simulink model "sim_att_dist_obs_tie_2025"  (R2020a)
settings: Solver=ode4  StartTime=0.0  StopTime=30.0  FixedStep=0.01  RelTol=1e-3
values from neighbouring files (symbols this model uses):
  beta_Phi_1 = pp0 * cal_frac_squ( 3, p_p0_plus_1, q_p0_plus_1 )                          * cal_frac_squ( eps_s_bar / pi, p_p0_min_2, q_p0_min_2 )                          / ( 2 * ( 2 * pp0 - 1 ) * tanh( gamma0 * ( eps_s_bar / pi ) / 2 ) )                          - ( cal_frac_squ( 3, p_p0_plus_1, q_p0_plus_1 ) * gamma0 / ( 4 * ( 2 * pp0 -1 ) ) )                          * cal_frac_squ( eps_s_bar / pi, p_p0_min_ ...(+136 chars)    [init_att_dist_obs_tie_2025.m]
  beta_Phi_2 = ( 1 - pp0 ) * cal_frac_squ( 3, p_p0_plus_1, q_p0_plus_1 )                          / ( 2 * ( 1 - 2 * pp0 ) * cal_frac_squ( eps_s_bar / pi, p_p0_0, q_p0_0 ) * tanh( gamma0 * ( eps_s_bar / pi ) / 2 ) )                          - ( cal_frac_squ( 3, p_p0_plus_1, q_p0_plus_1 ) * gamma0 / ( 4 * ( 1 - 2 * pp0 ) ) )                          * cal_frac_squ( eps_s_bar / pi, p_1_min_p0, q_1_min_p0 )          ...(+112 chars)    [init_att_dist_obs_tie_2025.m]
  c1_diff_ui = diag([25; 30; 20])    [init_att_dist_obs_tie_2025.m]
  c2_diff_ui = diag([50; 50; 10])    [init_att_dist_obs_tie_2025.m]
  c3_diff_ui = diag([15; 15; 10])    [init_att_dist_obs_tie_2025.m]
  c_w_1 = diag( [20; 15; 15] )    [init_att_dist_obs_tie_2025.m]
  c_w_2 = diag( [20; 15; 15] )    [init_att_dist_obs_tie_2025.m]
  c_w_3 = diag( [2; 2; 2] )    [init_att_dist_obs_tie_2025.m]
  cS0 = diag( [4.5; 4.5; 4.5] )    [init_att_dist_obs_tie_2025.m]
  dw_aa_t = 0.2 * ones(3, 5) + ( 1.0 - 0.2 ) * rand(3, 5)    [init_att_dist_obs_tie_2025.m]
  dw_ff_t = [ 0.4 * ones(1, 5) + ( 1.0 - 0.4 ) * rand(1, 5);                      0.4 * ones(1, 5) + ( 1.0 - 0.4 ) * rand(1, 5);                      0.2 * ones(1, 5) + ( 0.6 - 0.2 ) * rand(1, 5) ]    [init_att_dist_obs_tie_2025.m]
  dw_phi_t = ( - pi / 2 ) * ones(3, 5) + ( pi / 2 - ( - pi / 2 ) ) * rand(3, 5)    [init_att_dist_obs_tie_2025.m]
  dwci_init = zeros(3,5)    [init_att_dist_obs_tie_2025.m]
  eps_s_bar_div_pi = eps_s_bar / pi    (= 0.03)    [init_att_dist_obs_tie_2025.m]
  gamma0 = 20    [init_att_dist_obs_tie_2025.m]
  Ji = zeros(3,3,NF)    [init_att_dist_obs_tie_2025.m]
  k_J_0 = diag( [1; 1; 1] )    [init_att_dist_obs_tie_2025.m]
  lam1w = [40; 40; 40]    [init_att_dist_obs_tie_2025.m]
  lam2w = [50; 50; 50]    [init_att_dist_obs_tie_2025.m]
  Lamd_diff_ui = 0.8    [init_att_dist_obs_tie_2025.m]
  mu_c_theta = 100    [init_att_dist_obs_tie_2025.m]
  p1w = [1; 1; 1]    [init_att_dist_obs_tie_2025.m]
  pos0 = zeros(3, 1)    [init_att_dist_obs_tie_2025.m]
  pp0 = 8 / 11    (= 0.727272727273)    [init_att_dist_obs_tie_2025.m]
  PZ0 = P0(3)    [init_att_dist_obs_tie_2025.m]
  PZ1 = 10    [init_att_dist_obs_tie_2025.m]
  Qci_init = repmat([1;0;0;0],1,NF)    [init_att_dist_obs_tie_2025.m]
  R0 = 4    [init_att_dist_obs_tie_2025.m]
  R1 = 8    [init_att_dist_obs_tie_2025.m]
  Rci_init = zeros(3,3,NF)    [init_att_dist_obs_tie_2025.m]
  Ri_init = zeros(3,3,NF)    [init_att_dist_obs_tie_2025.m]
  Rx2 = 10    [init_att_dist_obs_tie_2025.m]
  Ry2 = 6    [init_att_dist_obs_tie_2025.m]
  Rz2 = 4    [init_att_dist_obs_tie_2025.m]
  T0 = 0    [init_att_dist_obs_tie_2025.m]
  T1 = tseq1    (= 10)    [init_att_dist_obs_tie_2025.m]
  T2 = tseq1 + tseq12 + tseq2    (= 30)    [init_att_dist_obs_tie_2025.m]
  thr_p_plus_1 = cal_frac_squ( 3, p_p0_plus_1, q_p0_plus_1 )    [init_att_dist_obs_tie_2025.m]
  ui_init = zeros(3,NF)    [init_att_dist_obs_tie_2025.m]
  vel0 = zeros(3, 1)    [init_att_dist_obs_tie_2025.m]
  wci_init = zeros(3,5)    [init_att_dist_obs_tie_2025.m]
  zeta_diff_ui = 0.05    [init_att_dist_obs_tie_2025.m]
undefined symbols (not defined in the file or in its folder): cal_frac_squ, p_2_mu, p_2_p0, p_2mu_1, p_3_2mu, p_beta_w_1, p_beta_w_2, p_mu, p_p0_min_1, p_p0_plus_1, q_2_mu, q_2_p0, q_2mu_1, q_3_2mu, q_beta_w_1, q_beta_w_2, q_mu, q_p0_min_1, q_p0_plus_1, Qei_init, Qi_init, Rei_init, V_Phi_Rei_init, wei_init, wi_init
(part 4 of 4)

== matlab function sim_att_dist_obs_tie_2025/generate angular rate disturbance agent 3 ==
  data: dw_3 output; dw_aa_t input; dw_ff_t input; dw_phi_t input; t input
function dw_3 = fcn(dw_aa_t, dw_ff_t, dw_phi_t, t)
%%%% 姿态动力学方程中的扰动项设置
epsil_t = zeros(3, 1);

for kk = 1:5
    epsil_t = epsil_t + dw_aa_t(:, kk) .* sin( 2 * pi * dw_ff_t(:, kk) * t + dw_phi_t(:, kk) );
end

dw_3 = [ epsil_t(1) + 1.6 * sin( 0.2 * t ) + 2.0 * cos( 0.3 * t ) + 1.4 * sin( 0.5 * t ) ...
                + 4 * exp( -0.1 * t ) * sin( 0.5 * t ) + 3 / ( 1 + exp( -0.2 * ( t - 15 ) ) ); ...
                epsil_t(2) + 1.2 * sin( 0.1 * t ) + 3 * cos( 0.2 * t ) + 0.8 * sin( 0.4 * t ) ...
                + 2 * exp( -0.15 * t ) * cos( 0.6 * t ) + 3 / ( 1 + exp( -0.3 * ( t - 25 ) ) ); ...
                epsil_t(3) + 1.8 * sin( 0.1 * t ) + 1.6 * sin( 0.2 * t ) + 1.6 * cos( 0.3 * t ) ...
                + 4 * exp( -0.05 * t ) * sin( 0.4 * t + pi / 4 ) + 3 / ( 1 + exp( -0.5 * ( t - 20 ) ) ) ];

== matlab function sim_att_dist_obs_tie_2025/generate angular rate disturbance agent 4 ==
  data: dw_4 output; dw_aa_t input; dw_ff_t input; dw_phi_t input; t input
function dw_4 = fcn(dw_aa_t, dw_ff_t, dw_phi_t, t)
%%%% 姿态动力学方程中的扰动项设置
epsil_t = zeros(3, 1);

for kk = 1:5
    epsil_t = epsil_t + dw_aa_t(:, kk) .* sin( 2 * pi * dw_ff_t(:, kk) * t + dw_phi_t(:, kk) );
end

dw_4 = [ epsil_t(1) + 1.6 * sin( 0.2 * t ) + 2.0 * cos( 0.3 * t ) + 1.4 * sin( 0.5 * t ) ...
                + 4 * exp( -0.1 * t ) * sin( 0.5 * t ) + 3 / ( 1 + exp( -0.2 * ( t - 15 ) ) ); ...
                epsil_t(2) + 1.2 * sin( 0.1 * t ) + 3 * cos( 0.2 * t ) + 0.8 * sin( 0.4 * t ) ...
                + 2 * exp( -0.15 * t ) * cos( 0.6 * t ) + 3 / ( 1 + exp( -0.3 * ( t - 25 ) ) ); ...
                epsil_t(3) + 1.8 * sin( 0.1 * t ) + 1.6 * sin( 0.2 * t ) + 1.6 * cos( 0.3 * t ) ...
                + 4 * exp( -0.05 * t ) * sin( 0.4 * t + pi / 4 ) + 3 / ( 1 + exp( -0.5 * ( t - 20 ) ) ) ];

== matlab function sim_att_dist_obs_tie_2025/trans to column56 ==
  data: x input; y output
function y = fcn(x)
y = x(:);

== matlab function sim_att_dist_obs_tie_2025/generate angular rate disturbance agent 5 ==
  data: dw_5 output; dw_aa_t input; dw_ff_t input; dw_phi_t input; t input
function dw_5 = fcn(dw_aa_t, dw_ff_t, dw_phi_t, t)
%%%% 姿态动力学方程中的扰动项设置
epsil_t = zeros(3, 1);

for kk = 1:5
    epsil_t = epsil_t + dw_aa_t(:, kk) .* sin( 2 * pi * dw_ff_t(:, kk) * t + dw_phi_t(:, kk) );
end

dw_5 = [ epsil_t(1) + 1.6 * sin( 0.2 * t ) + 2.0 * cos( 0.3 * t ) + 1.4 * sin( 0.5 * t ) ...
                + 4 * exp( -0.1 * t ) * sin( 0.5 * t ) + 3 / ( 1 + exp( -0.2 * ( t - 15 ) ) ); ...
                epsil_t(2) + 1.2 * sin( 0.1 * t ) + 3 * cos( 0.2 * t ) + 0.8 * sin( 0.4 * t ) ...
                + 2 * exp( -0.15 * t ) * cos( 0.6 * t ) + 3 / ( 1 + exp( -0.3 * ( t - 25 ) ) ); ...
                epsil_t(3) + 1.8 * sin( 0.1 * t ) + 1.6 * sin( 0.2 * t ) + 1.6 * cos( 0.3 * t ) ...
                + 4 * exp( -0.05 * t ) * sin( 0.4 * t + pi / 4 ) + 3 / ( 1 + exp( -0.5 * ( t - 20 ) ) ) ];

== matlab function sim_att_dist_obs_tie_2025/trans to column100 ==
  data: x input; y output
function y = fcn(x)
y = x(:);

== matlab function sim_att_dist_obs_tie_2025/trans to column101 ==
  data: x input; y output
function y = fcn(x)
y = x(:);

== matlab function sim_att_dist_obs_tie_2025/trans to column102 ==
  data: x input; y output
function y = fcn(x)
y = x(:);

== matlab function sim_att_dist_obs_tie_2025/trans to column103 ==
  data: x input; y output
function y = fcn(x)
y = x(:);

== matlab function sim_att_dist_obs_tie_2025/trans to column104 ==
  data: x input; y output
function y = fcn(x)
y = x(:);

== matlab function sim_att_dist_obs_tie_2025/trans to column105 ==
  data: x input; y output
function y = fcn(x)
y = x(:);

== matlab function sim_att_dist_obs_tie_2025/trans to column106 ==
  data: x input; y output
function y = fcn(x)
y = x(:);

== matlab function sim_att_dist_obs_tie_2025/trans to column116 ==
  data: x input; y output
function y = fcn(x)
y = x(:);

== matlab function sim_att_dist_obs_tie_2025/cal abs 17 ==
  data: x input; y output
function y = fcn(x)
y = abs(x(:));

== matlab function sim_att_dist_obs_tie_2025/trans to column118 ==
  data: x input; y output
function y = fcn(x)
y = x(:);

== matlab function sim_att_dist_obs_tie_2025/trans to column119 ==
  data: x input; y output
function y = fcn(x)
y = x(:);

== matlab function sim_att_dist_obs_tie_2025/trans to column120 ==
  data: x input; y output
function y = fcn(x)
y = x(:);

== matlab function sim_att_dist_obs_tie_2025/trans to column121 ==
  data: x input; y output
function y = fcn(x)
y = x(:);

== matlab function sim_att_dist_obs_tie_2025/trans to column122 ==
  data: x input; y output
function y = fcn(x)
y = x(:);

== matlab function sim_att_dist_obs_tie_2025/trans to column123 ==
  data: x input; y output
function y = fcn(x)
y = x(:);

== matlab function sim_att_dist_obs_tie_2025/trans to column124 ==
  data: x input; y output
function y = fcn(x)
y = x(:);

== matlab function sim_att_dist_obs_tie_2025/trans to column125 ==
  data: x input; y output
function y = fcn(x)
y = x(:);

== matlab function sim_att_dist_obs_tie_2025/trans to column61 ==
  data: x input; y output
function y = fcn(x)
y = x(:);

== matlab function sim_att_dist_obs_tie_2025/trans to column62 ==
  data: x input; y output
function y = fcn(x)
y = x(:);

== matlab function sim_att_dist_obs_tie_2025/cal abs 18 ==
  data: x input; y output
function y = fcn(x)
y = abs(x(:));

== matlab function sim_att_dist_obs_tie_2025/trans to column63 ==
  data: x input; y output
function y = fcn(x)
y = x(:);

== matlab function sim_att_dist_obs_tie_2025/trans to column64 ==
  data: x input; y output
function y = fcn(x)
y = x(:);

== matlab function sim_att_dist_obs_tie_2025/trans to column65 ==
  data: x input; y output
function y = fcn(x)
y = x(:);

== matlab function sim_att_dist_obs_tie_2025/trans to column66 ==
  data: x input; y output
function y = fcn(x)
y = x(:);

== matlab function sim_att_dist_obs_tie_2025/trans to column67 ==
  data: x input; y output
function y = fcn(x)
y = x(:);

== matlab function sim_att_dist_obs_tie_2025/trans to column68 ==
  data: x input; y output
function y = fcn(x)
y = x(:);

== matlab function sim_att_dist_obs_tie_2025/trans to column69 ==
  data: x input; y output
function y = fcn(x)
y = x(:);

== matlab function sim_att_dist_obs_tie_2025/trans to column70 ==
  data: x input; y output
function y = fcn(x)
y = x(:);

== matlab function sim_att_dist_obs_tie_2025/trans to column71 ==
  data: x input; y output
function y = fcn(x)
y = x(:);

== matlab function sim_att_dist_obs_tie_2025/trans to column72 ==
  data: x input; y output
function y = fcn(x)
y = x(:);

== matlab function sim_att_dist_obs_tie_2025/cal sig_x1_tilt agent 4 ==
  data: sig_x1_tilt_1_4 output; x1_tilt_vec input; x1_tilt_squ_1_4 input; sig_x1_tilt_2_4 output; x1_tilt_squ_2_4 input; sig_x1_tilt_3_4 output
function [sig_x1_tilt_1_4, sig_x1_tilt_2_4, sig_x1_tilt_3_4] = fcn(x1_tilt_vec, x1_tilt_squ_1_4, x1_tilt_squ_2_4)
%%%% 计算平滑递增函数
iiuav = 4;
sig_x1_tilt_1_4 = x1_tilt_vec(:,iiuav) .* sign(x1_tilt_vec(:,iiuav));
sig_x1_tilt_2_4 = x1_tilt_squ_1_4(:) .* sign(x1_tilt_vec(:,iiuav));
sig_x1_tilt_3_4 = x1_tilt_squ_2_4(:) .* sign(x1_tilt_vec(:,iiuav));

== matlab function sim_att_dist_obs_tie_2025/trans to column73 ==
  data: x input; y output
function y = fcn(x)
y = x(:);

== matlab function sim_att_dist_obs_tie_2025/trans to column74 ==
  data: x input; y output
function y = fcn(x)
y = x(:);

== matlab function sim_att_dist_obs_tie_2025/trans to column75 ==
  data: x input; y output
function y = fcn(x)
y = x(:);

== matlab function sim_att_dist_obs_tie_2025/trans to column76 ==
  data: x input; y output
function y = fcn(x)
y = x(:);

== matlab function sim_att_dist_obs_tie_2025/trans to column77 ==
  data: x input; y output
function y = fcn(x)
y = x(:);

== matlab function sim_att_dist_obs_tie_2025/trans to column78 ==
  data: x input; y output
function y = fcn(x)
y = x(:);

== matlab function sim_att_dist_obs_tie_2025/trans to column79 ==
  data: x input; y output
function y = fcn(x)
y = x(:);

== matlab function sim_att_dist_obs_tie_2025/trans to column80 ==
  data: x input; y output
function y = fcn(x)
y = x(:);

== matlab function sim_att_dist_obs_tie_2025/trans to column81 ==
  data: x input; y output
function y = fcn(x)
y = x(:);

== matlab function sim_att_dist_obs_tie_2025/trans to column82 ==
  data: x input; y output
function y = fcn(x)
y = x(:);

== matlab function sim_att_dist_obs_tie_2025/trans to column83 ==
  data: x input; y output
function y = fcn(x)
y = x(:);

== matlab function sim_att_dist_obs_tie_2025/trans to column84 ==
  data: x input; y output
function y = fcn(x)
y = x(:);

== matlab function sim_att_dist_obs_tie_2025/trans to column85 ==
  data: x input; y output
function y = fcn(x)
y = x(:);

== matlab function sim_att_dist_obs_tie_2025/trans to column86 ==
  data: x input; y output
function y = fcn(x)
y = x(:);

== matlab function sim_att_dist_obs_tie_2025/trans to column87 ==
  data: x input; y output
function y = fcn(x)
y = x(:);

== matlab function sim_att_dist_obs_tie_2025/trans to column88 ==
  data: x input; y output
function y = fcn(x)
y = x(:);

== matlab function sim_att_dist_obs_tie_2025/choose ksi_est_err 17 ==
  data: x input; y output
function y = fcn(x)
iiuav = 4;
y = x(:,iiuav);

== matlab function sim_att_dist_obs_tie_2025/trans to column89 ==
  data: x input; y output
function y = fcn(x)
y = x(:);

== matlab function sim_att_dist_obs_tie_2025/trans to column90 ==
  data: x input; y output
function y = fcn(x)
y = x(:);

== matlab function sim_att_dist_obs_tie_2025/trans to column91 ==
  data: x input; y output
function y = fcn(x)
y = x(:);

== matlab function sim_att_dist_obs_tie_2025/trans to column92 ==
  data: x input; y output
function y = fcn(x)
y = x(:);

== matlab function sim_att_dist_obs_tie_2025/trans to column93 ==
  data: x input; y output
function y = fcn(x)
y = x(:);

== matlab function sim_att_dist_obs_tie_2025/trans to column94 ==
  data: x input; y output
function y = fcn(x)
y = x(:);

== matlab function sim_att_dist_obs_tie_2025/trans to column95 ==
  data: x input; y output
function y = fcn(x)
y = x(:);

== matlab function sim_att_dist_obs_tie_2025/trans to column96 ==
  data: x input; y output
function y = fcn(x)
y = x(:);

== matlab function sim_att_dist_obs_tie_2025/trans to column97 ==
  data: x input; y output
function y = fcn(x)
y = x(:);

== matlab function sim_att_dist_obs_tie_2025/trans to column98 ==
  data: x input; y output
function y = fcn(x)
y = x(:);

== matlab function sim_att_dist_obs_tie_2025/choose ksi_est_err 18 ==
  data: x input; y output
function y = fcn(x)
iiuav = 4;
y = x(:,iiuav);

== matlab function sim_att_dist_obs_tie_2025/trans to column99 ==
  data: x input; y output
function y = fcn(x)
y = x(:);

== matlab function sim_att_dist_obs_tie_2025/wi dynam agent 1 ==
  data: Ji input; dwi_1 output; wi_vec input; taui_vec input; dw_vec input
function dwi_1 = fcn(Ji, wi_vec, taui_vec, dw_vec)
%%%% 更新姿态角速率微分方程
iiuav = 1;
dwi_1 = inv(Ji(:,:,iiuav)) * ( -cal_askew_mat(wi_vec(:,iiuav)) * Ji(:,:,iiuav) * wi_vec(:,iiuav) ... 
                                                + taui_vec(:,iiuav) + dw_vec(:,iiuav) );

end

== matlab function sim_att_dist_obs_tie_2025/wi dynam agent 2 ==
  data: Ji input; dwi_2 output; wi_vec input; taui_vec input; dw_vec input
function dwi_2 = fcn(Ji, wi_vec, taui_vec, dw_vec)
%%%% 更新姿态角速率微分方程
iiuav = 2;
dwi_2 = inv(Ji(:,:,iiuav)) * ( -cal_askew_mat(wi_vec(:,iiuav)) * Ji(:,:,iiuav) * wi_vec(:,iiuav) ... 
                                                + taui_vec(:,iiuav) + dw_vec(:,iiuav) );

end

== matlab function sim_att_dist_obs_tie_2025/wi dynam agent 3 ==
  data: Ji input; dwi_3 output; wi_vec input; taui_vec input; dw_vec input
function dwi_3 = fcn(Ji, wi_vec, taui_vec, dw_vec)
%%%% 更新姿态角速率微分方程
iiuav = 3;
dwi_3 = inv(Ji(:,:,iiuav)) * ( -cal_askew_mat(wi_vec(:,iiuav)) * Ji(:,:,iiuav) * wi_vec(:,iiuav) ...
                                                + taui_vec(:,iiuav) + dw_vec(:,iiuav) );

end

== matlab function sim_att_dist_obs_tie_2025/wi dynam agent 4 ==
  data: Ji input; dwi_4 output; wi_vec input; taui_vec input; dw_vec input
function dwi_4 = fcn(Ji, wi_vec, taui_vec, dw_vec)
%%%% 更新姿态角速率微分方程
iiuav = 4;
dwi_4 = inv(Ji(:,:,iiuav)) * ( -cal_askew_mat(wi_vec(:,iiuav)) * Ji(:,:,iiuav) * wi_vec(:,iiuav) ...
                                                + taui_vec(:,iiuav) + dw_vec(:,iiuav) );

end

== matlab function sim_att_dist_obs_tie_2025/wi dynam agent 5 ==
  data: Ji input; dwi_5 output; wi_vec input; taui_vec input; dw_vec input
function dwi_5 = fcn(Ji, wi_vec, taui_vec, dw_vec)
%%%% 更新姿态角速率微分方程
iiuav = 5;
dwi_5 = inv(Ji(:,:,iiuav)) * ( -cal_askew_mat(wi_vec(:,iiuav)) * Ji(:,:,iiuav) * wi_vec(:,iiuav) ...
                                                + taui_vec(:,iiuav) + dw_vec(:,iiuav) );

end

== matlab function sim_att_dist_obs_tie_2025/combine norminal formation control input ==
  data: ui_1 input; ui_vec output; ui_2 input; ui_3 input; ui_4 input; ui_5 input
function ui_vec = fcn(ui_1, ui_2, ui_3, ui_4, ui_5)
%%%% 合并领导者编队跟踪误差结果
ui_vec = [ui_1(:), ui_2(:), ui_3(:), ui_4(:), ui_5(:)];

== matlab function sim_att_dist_obs_tie_2025/trans to column57 ==
  data: x input; y output
function y = fcn(x)
y = x(:);

== matlab function sim_att_dist_obs_tie_2025/control input generator agent 1 ==
  data: u0 input; ui output
function ui  = fcn(u0)
%%%% 给出领导者参考加速度控制输入
g0 = 9.80663;
e3 = [0;0;1];

ui = g0 * e3 + u0(:);

== matlab function sim_att_dist_obs_tie_2025/control input generator agent 2 ==
  data: u0 input; ui output
function ui  = fcn(u0)
%%%% 给出领导者参考加速度控制输入
g0 = 9.80663;
e3 = [0;0;1];

ui = g0 * e3 + u0(:);

== matlab function sim_att_dist_obs_tie_2025/control input generator agent 3 ==
  data: u0 input; ui output
function ui  = fcn(u0)
%%%% 给出领导者参考加速度控制输入
g0 = 9.80663;
e3 = [0;0;1];

ui = g0 * e3 + u0(:);

== matlab function sim_att_dist_obs_tie_2025/control input generator agent 4 ==
  data: u0 input; ui output
function ui  = fcn(u0)
%%%% 给出领导者参考加速度控制输入
g0 = 9.80663;
e3 = [0;0;1];

ui = g0 * e3 + u0(:);

== matlab function sim_att_dist_obs_tie_2025/control input generator agent 5 ==
  data: u0 input; ui output
function ui  = fcn(u0)
%%%% 给出领导者参考加速度控制输入
g0 = 9.80663;
e3 = [0;0;1];

ui = g0 * e3 + u0(:);

== matlab function sim_att_dist_obs_tie_2025/trans to column58 ==
  data: x input; y output
function y = fcn(x)
y = x(:);

== matlab function sim_att_dist_obs_tie_2025/cal abs 19 ==
  data: x input; y output
function y = fcn(x)
y = abs(x(:));

== matlab function sim_att_dist_obs_tie_2025/cal abs 20 ==
  data: x input; y output
function y = fcn(x)
y = abs(x(:));

== matlab function sim_att_dist_obs_tie_2025/cal sig_x1_tilt agent 5 ==
  data: sig_x1_tilt_1_5 output; x1_tilt_vec input; x1_tilt_squ_1_5 input; sig_x1_tilt_2_5 output; x1_tilt_squ_2_5 input; sig_x1_tilt_3_5 output
function [sig_x1_tilt_1_5, sig_x1_tilt_2_5, sig_x1_tilt_3_5] = fcn(x1_tilt_vec, x1_tilt_squ_1_5, x1_tilt_squ_2_5)
%%%% 计算平滑递增函数
iiuav = 5;
sig_x1_tilt_1_5 = x1_tilt_vec(:,iiuav) .* sign(x1_tilt_vec(:,iiuav));
sig_x1_tilt_2_5 = x1_tilt_squ_1_5(:) .* sign(x1_tilt_vec(:,iiuav));
sig_x1_tilt_3_5 = x1_tilt_squ_2_5(:) .* sign(x1_tilt_vec(:,iiuav));

== matlab function sim_att_dist_obs_tie_2025/choose ksi_est_err 19 ==
  data: x input; y output
function y = fcn(x)
iiuav = 5;
y = x(:,iiuav);

== matlab function sim_att_dist_obs_tie_2025/choose ksi_est_err 20 ==
  data: x input; y output
function y = fcn(x)
iiuav = 5;
y = x(:,iiuav);

== matlab function sim_att_dist_obs_tie_2025/trans to column59 ==
  data: x input; y output
function y = fcn(x)
y = x(:);

== matlab function sim_att_dist_obs_tie_2025/trans to column60 ==
  data: x input; y output
function y = fcn(x)
y = x(:);

== matlab function sim_att_dist_obs_tie_2025/cal x1_hat agent 1 ==
  data: d_x1_hat_1 output; Ji input; lam1w input; wi_vec input; taui_vec input; dw_hat_vec input; sig_x1_tilt_1_vec input; sig_x1_tilt_2_vec input; sig_x1_tilt_3_vec input
function d_x1_hat_1 = fcn(Ji, lam1w, wi_vec, taui_vec, dw_hat_vec, sig_x1_tilt_1_vec, sig_x1_tilt_2_vec, sig_x1_tilt_3_vec)
%%%% 计算平滑递增函数
iiuav = 1;
d_x1_hat_1 = -cal_askew_mat(wi_vec(:,iiuav)) * Ji(:,:,iiuav) * wi_vec(:,iiuav) + taui_vec(:,iiuav) ...
                            + dw_hat_vec(:,iiuav) + lam1w(:) .* (sig_x1_tilt_1_vec(:,iiuav) + sig_x1_tilt_2_vec(:,iiuav) + sig_x1_tilt_3_vec(:,iiuav));

== matlab function sim_att_dist_obs_tie_2025/cal x1_hat agent 2 ==
  data: d_x1_hat_2 output; Ji input; lam1w input; wi_vec input; taui_vec input; dw_hat_vec input; sig_x1_tilt_1_vec input; sig_x1_tilt_2_vec input; sig_x1_tilt_3_vec input
function d_x1_hat_2 = fcn(Ji, lam1w, wi_vec, taui_vec, dw_hat_vec, sig_x1_tilt_1_vec, sig_x1_tilt_2_vec, sig_x1_tilt_3_vec)
%%%% 计算平滑递增函数
iiuav = 2;
d_x1_hat_2 = -cal_askew_mat(wi_vec(:,iiuav)) * Ji(:,:,iiuav) * wi_vec(:,iiuav) + taui_vec(:,iiuav) ...
                            + dw_hat_vec(:,iiuav) + lam1w(:) .* (sig_x1_tilt_1_vec(:,iiuav) + sig_x1_tilt_2_vec(:,iiuav) + sig_x1_tilt_3_vec(:,iiuav));

== matlab function sim_att_dist_obs_tie_2025/cal x1_hat agent 3 ==
  data: d_x1_hat_3 output; Ji input; lam1w input; wi_vec input; taui_vec input; dw_hat_vec input; sig_x1_tilt_1_vec input; sig_x1_tilt_2_vec input; sig_x1_tilt_3_vec input
function d_x1_hat_3 = fcn(Ji, lam1w, wi_vec, taui_vec, dw_hat_vec, sig_x1_tilt_1_vec, sig_x1_tilt_2_vec, sig_x1_tilt_3_vec)
%%%% 计算平滑递增函数
iiuav = 3;
d_x1_hat_3 = -cal_askew_mat(wi_vec(:,iiuav)) * Ji(:,:,iiuav) * wi_vec(:,iiuav) + taui_vec(:,iiuav) ...
                            + dw_hat_vec(:,iiuav) + lam1w(:) .* (sig_x1_tilt_1_vec(:,iiuav) + sig_x1_tilt_2_vec(:,iiuav) + sig_x1_tilt_3_vec(:,iiuav));

== matlab function sim_att_dist_obs_tie_2025/cal x1_hat agent 4 ==
  data: d_x1_hat_4 output; Ji input; lam1w input; wi_vec input; taui_vec input; dw_hat_vec input; sig_x1_tilt_1_vec input; sig_x1_tilt_2_vec input; sig_x1_tilt_3_vec input
function d_x1_hat_4 = fcn(Ji, lam1w, wi_vec, taui_vec, dw_hat_vec, sig_x1_tilt_1_vec, sig_x1_tilt_2_vec, sig_x1_tilt_3_vec)
%%%% 计算平滑递增函数
iiuav = 4;
d_x1_hat_4 = -cal_askew_mat(wi_vec(:,iiuav)) * Ji(:,:,iiuav) * wi_vec(:,iiuav) + taui_vec(:,iiuav) ...
                            + dw_hat_vec(:,iiuav) + lam1w(:) .* (sig_x1_tilt_1_vec(:,iiuav) + sig_x1_tilt_2_vec(:,iiuav) + sig_x1_tilt_3_vec(:,iiuav));

== matlab function sim_att_dist_obs_tie_2025/cal x1_hat agent 5 ==
  data: d_x1_hat_5 output; Ji input; lam1w input; wi_vec input; taui_vec input; dw_hat_vec input; sig_x1_tilt_1_vec input; sig_x1_tilt_2_vec input; sig_x1_tilt_3_vec input
function d_x1_hat_5 = fcn(Ji, lam1w, wi_vec, taui_vec, dw_hat_vec, sig_x1_tilt_1_vec, sig_x1_tilt_2_vec, sig_x1_tilt_3_vec)
%%%% 计算平滑递增函数
iiuav = 5;
d_x1_hat_5 = -cal_askew_mat(wi_vec(:,iiuav)) * Ji(:,:,iiuav) * wi_vec(:,iiuav) + taui_vec(:,iiuav) ...
                            + dw_hat_vec(:,iiuav) + lam1w(:) .* (sig_x1_tilt_1_vec(:,iiuav) + sig_x1_tilt_2_vec(:,iiuav) + sig_x1_tilt_3_vec(:,iiuav));

== matlab function sim_att_dist_obs_tie_2025/cal abs 31 ==
  data: x input; y output
function y = fcn(x)
y = abs(x(:));

== matlab function sim_att_dist_obs_tie_2025/cal abs 32 ==
  data: x input; y output
function y = fcn(x)
y = abs(x(:));

== matlab function sim_att_dist_obs_tie_2025/cal abs 33 ==
  data: x input; y output
function y = fcn(x)
y = abs(x(:));

== matlab function sim_att_dist_obs_tie_2025/cal abs 34 ==
  data: x input; y output
function y = fcn(x)
y = abs(x(:));

== matlab function sim_att_dist_obs_tie_2025/cal sig_x1_tilt other agent 2 ==
  data: sig_x1_tilt_4_2 output; x1_tilt_vec input; x1_tilt_squ_4_2 input; sig_x1_tilt_5_2 output; x1_tilt_squ_5_2 input
function [sig_x1_tilt_4_2, sig_x1_tilt_5_2] = fcn(x1_tilt_vec, x1_tilt_squ_4_2, x1_tilt_squ_5_2)
%%%% 计算平滑递增函数
iiuav = 2;
sig_x1_tilt_4_2 = x1_tilt_squ_4_2(:) .* sign(x1_tilt_vec(:,iiuav));
sig_x1_tilt_5_2 = x1_tilt_squ_5_2(:) .* sign(x1_tilt_vec(:,iiuav));

== matlab function sim_att_dist_obs_tie_2025/choose ksi_est_err 33 ==
  data: x input; y output
function y = fcn(x)
iiuav = 2;
y = x(:,iiuav);

== matlab function sim_att_dist_obs_tie_2025/choose ksi_est_err 34 ==
  data: x input; y output
function y = fcn(x)
iiuav = 2;
y = x(:,iiuav);

== matlab function sim_att_dist_obs_tie_2025/trans to column3 ==
  data: x input; y output
function y = fcn(x)
y = x(:);

== matlab function sim_att_dist_obs_tie_2025/trans to column4 ==
  data: x input; y output
function y = fcn(x)
y = x(:);

== matlab function sim_att_dist_obs_tie_2025/cal abs 35 ==
  data: x input; y output
function y = fcn(x)
y = abs(x(:));

== matlab function sim_att_dist_obs_tie_2025/cal abs 36 ==
  data: x input; y output
function y = fcn(x)
y = abs(x(:));

== matlab function sim_att_dist_obs_tie_2025/cal x1_tilt ==
  data: Ji input; p1w input; x1_tilt_vec output; wi_vec input; x1_hat_vec input
function x1_tilt_vec = fcn(Ji, p1w, wi_vec, x1_hat_vec)
%%%% 计算姿态角速率观测误差
x1_tilt_vec = zeros(3,5);
for iiuav = 1:5
    x1_tilt_vec(:,iiuav) = (1 ./ p1w) .* ( Ji(:,:,iiuav) * wi_vec(:,iiuav) - x1_hat_vec(:,iiuav) );
end

== matlab function sim_att_dist_obs_tie_2025/cal sig_x1_tilt other agent 1 ==
  data: sig_x1_tilt_4_1 output; x1_tilt_vec input; x1_tilt_squ_4_1 input; sig_x1_tilt_5_1 output; x1_tilt_squ_5_1 input
function [sig_x1_tilt_4_1, sig_x1_tilt_5_1] = fcn(x1_tilt_vec, x1_tilt_squ_4_1, x1_tilt_squ_5_1)
%%%% 计算平滑递增函数
iiuav = 1;
sig_x1_tilt_4_1 = x1_tilt_squ_4_1(:) .* sign(x1_tilt_vec(:,iiuav));
sig_x1_tilt_5_1 = x1_tilt_squ_5_1(:) .* sign(x1_tilt_vec(:,iiuav));

== matlab function sim_att_dist_obs_tie_2025/cal sig_x1_tilt other agent 3 ==
  data: sig_x1_tilt_4_3 output; x1_tilt_vec input; x1_tilt_squ_4_3 input; sig_x1_tilt_5_3 output; x1_tilt_squ_5_3 input
function [sig_x1_tilt_4_3, sig_x1_tilt_5_3] = fcn(x1_tilt_vec, x1_tilt_squ_4_3, x1_tilt_squ_5_3)
%%%% 计算平滑递增函数
iiuav = 3;
sig_x1_tilt_4_3 = x1_tilt_squ_4_3(:) .* sign(x1_tilt_vec(:,iiuav));
sig_x1_tilt_5_3 = x1_tilt_squ_5_3(:) .* sign(x1_tilt_vec(:,iiuav));

== matlab function sim_att_dist_obs_tie_2025/choose ksi_est_err 35 ==
  data: x input; y output
function y = fcn(x)
iiuav = 3;
y = x(:,iiuav);

== matlab function sim_att_dist_obs_tie_2025/choose ksi_est_err 36 ==
  data: x input; y output
function y = fcn(x)
iiuav = 3;
y = x(:,iiuav);

== matlab function sim_att_dist_obs_tie_2025/choose ksi_est_err 31 ==
  data: x input; y output
function y = fcn(x)
iiuav = 1;
y = x(:,iiuav);

== matlab function sim_att_dist_obs_tie_2025/choose ksi_est_err 32 ==
  data: x input; y output
function y = fcn(x)
iiuav = 1;
y = x(:,iiuav);

== matlab function sim_att_dist_obs_tie_2025/trans to column5 ==
  data: x input; y output
function y = fcn(x)
y = x(:);

== matlab function sim_att_dist_obs_tie_2025/trans to column6 ==
  data: x input; y output
function y = fcn(x)
y = x(:);

== matlab function sim_att_dist_obs_tie_2025/cal abs 37 ==
  data: x input; y output
function y = fcn(x)
y = abs(x(:));

== matlab function sim_att_dist_obs_tie_2025/cal abs 38 ==
  data: x input; y output
function y = fcn(x)
y = abs(x(:));

== matlab function sim_att_dist_obs_tie_2025/cal sig_x1_tilt other agent 4 ==
  data: sig_x1_tilt_4_4 output; x1_tilt_vec input; x1_tilt_squ_4_4 input; sig_x1_tilt_5_4 output; x1_tilt_squ_5_4 input
function [sig_x1_tilt_4_4, sig_x1_tilt_5_4] = fcn(x1_tilt_vec, x1_tilt_squ_4_4, x1_tilt_squ_5_4)
%%%% 计算平滑递增函数
iiuav = 4;
sig_x1_tilt_4_4 = x1_tilt_squ_4_4(:) .* sign(x1_tilt_vec(:,iiuav));
sig_x1_tilt_5_4 = x1_tilt_squ_5_4(:) .* sign(x1_tilt_vec(:,iiuav));

== matlab function sim_att_dist_obs_tie_2025/choose ksi_est_err 37 ==
  data: x input; y output
function y = fcn(x)
iiuav = 4;
y = x(:,iiuav);

== matlab function sim_att_dist_obs_tie_2025/choose ksi_est_err 38 ==
  data: x input; y output
function y = fcn(x)
iiuav = 4;
y = x(:,iiuav);

== matlab function sim_att_dist_obs_tie_2025/trans to column7 ==
  data: x input; y output
function y = fcn(x)
y = x(:);

== matlab function sim_att_dist_obs_tie_2025/combine sig_x1_tilt other ==
  data: sig_x1_tilt_4_1 input; sig_x1_tilt_4_2 input; sig_x1_tilt_4_3 input; sig_x1_tilt_4_4 input; sig_x1_tilt_4_5 input; sig_x1_tilt_4_vec output; sig_x1_tilt_5_1 input; sig_x1_tilt_5_vec output; sig_x1_tilt_5_2 input; sig_x1_tilt_5_3 input; sig_x1_tilt_5_4 input; sig_x1_tilt_5_5 input
function [sig_x1_tilt_4_vec, sig_x1_tilt_5_vec]  = fcn(sig_x1_tilt_4_1, sig_x1_tilt_4_2, sig_x1_tilt_4_3, sig_x1_tilt_4_4, sig_x1_tilt_4_5, ...
                                                                                                                                sig_x1_tilt_5_1, sig_x1_tilt_5_2, sig_x1_tilt_5_3, sig_x1_tilt_5_4, sig_x1_tilt_5_5)
%%%% 合并领导者位置观测器输出结果
sig_x1_tilt_4_vec = [sig_x1_tilt_4_1(:), sig_x1_tilt_4_2(:), sig_x1_tilt_4_3(:), sig_x1_tilt_4_4(:), sig_x1_tilt_4_5(:)];
sig_x1_tilt_5_vec = [sig_x1_tilt_5_1(:), sig_x1_tilt_5_2(:), sig_x1_tilt_5_3(:), sig_x1_tilt_5_4(:), sig_x1_tilt_5_5(:)];

== matlab function sim_att_dist_obs_tie_2025/trans to column1 ==
  data: x input; y output
function y = fcn(x)
y = x(:);

== matlab function sim_att_dist_obs_tie_2025/trans to column2 ==
  data: x input; y output
function y = fcn(x)
y = x(:);

== matlab function sim_att_dist_obs_tie_2025/trans to column8 ==
  data: x input; y output
function y = fcn(x)
y = x(:);

== matlab function sim_att_dist_obs_tie_2025/cal abs 39 ==
  data: x input; y output
function y = fcn(x)
y = abs(x(:));

== matlab function sim_att_dist_obs_tie_2025/cal abs 40 ==
  data: x input; y output
function y = fcn(x)
y = abs(x(:));

== matlab function sim_att_dist_obs_tie_2025/cal sig_x1_tilt other agent 5 ==
  data: sig_x1_tilt_4_5 output; x1_tilt_vec input; x1_tilt_squ_4_5 input; sig_x1_tilt_5_5 output; x1_tilt_squ_5_5 input
function [sig_x1_tilt_4_5, sig_x1_tilt_5_5] = fcn(x1_tilt_vec, x1_tilt_squ_4_5, x1_tilt_squ_5_5)
%%%% 计算平滑递增函数
iiuav = 5;
sig_x1_tilt_4_5 = x1_tilt_squ_4_5(:) .* sign(x1_tilt_vec(:,iiuav));
sig_x1_tilt_5_5 = x1_tilt_squ_5_5(:) .* sign(x1_tilt_vec(:,iiuav));

== matlab function sim_att_dist_obs_tie_2025/choose ksi_est_err 39 ==
  data: x input; y output
function y = fcn(x)
iiuav = 5;
y = x(:,iiuav);

== matlab function sim_att_dist_obs_tie_2025/choose ksi_est_err 40 ==
  data: x input; y output
function y = fcn(x)
iiuav = 5;
y = x(:,iiuav);

== matlab function sim_att_dist_obs_tie_2025/trans to column9 ==
  data: x input; y output
function y = fcn(x)
y = x(:);

== matlab function sim_att_dist_obs_tie_2025/trans to column10 ==
  data: x input; y output
function y = fcn(x)
y = x(:);

== matlab function sim_att_dist_obs_tie_2025/cal neso dw_hat agent 2 ==
  data: lam2w input; p1w input; sig_x1_tilt_1_vec input; sig_x1_tilt_4_vec input; sig_x1_tilt_5_vec input; d_dw_hat_2 output
function d_dw_hat_2 = fcn(lam2w, p1w, sig_x1_tilt_1_vec, sig_x1_tilt_4_vec, sig_x1_tilt_5_vec)
%%%% 计算扰动观测值
iiuav = 2;
d_dw_hat_2 = (lam2w(:) ./ p1w(:)) .* (sig_x1_tilt_1_vec(:,iiuav) + sig_x1_tilt_4_vec(:,iiuav) + sig_x1_tilt_5_vec(:,iiuav));

== matlab function sim_att_dist_obs_tie_2025/cal neso dw_hat agent 3 ==
  data: lam2w input; p1w input; sig_x1_tilt_1_vec input; sig_x1_tilt_4_vec input; sig_x1_tilt_5_vec input; d_dw_hat_3 output
function d_dw_hat_3 = fcn(lam2w, p1w, sig_x1_tilt_1_vec, sig_x1_tilt_4_vec, sig_x1_tilt_5_vec)
%%%% 计算扰动观测值
iiuav = 3;
d_dw_hat_3 = (lam2w(:) ./ p1w(:)) .* (sig_x1_tilt_1_vec(:,iiuav) + sig_x1_tilt_4_vec(:,iiuav) + sig_x1_tilt_5_vec(:,iiuav));

== matlab function sim_att_dist_obs_tie_2025/cal neso dw_hat agent 4 ==
  data: lam2w input; p1w input; sig_x1_tilt_1_vec input; sig_x1_tilt_4_vec input; sig_x1_tilt_5_vec input; d_dw_hat_4 output
function d_dw_hat_4 = fcn(lam2w, p1w, sig_x1_tilt_1_vec, sig_x1_tilt_4_vec, sig_x1_tilt_5_vec)
%%%% 计算扰动观测值
iiuav = 4;
d_dw_hat_4 = (lam2w(:) ./ p1w(:)) .* (sig_x1_tilt_1_vec(:,iiuav) + sig_x1_tilt_4_vec(:,iiuav) + sig_x1_tilt_5_vec(:,iiuav));

== matlab function sim_att_dist_obs_tie_2025/cal neso dw_hat agent 5 ==
  data: lam2w input; p1w input; sig_x1_tilt_1_vec input; sig_x1_tilt_4_vec input; sig_x1_tilt_5_vec input; d_dw_hat_5 output
function d_dw_hat_5 = fcn(lam2w, p1w, sig_x1_tilt_1_vec, sig_x1_tilt_4_vec, sig_x1_tilt_5_vec)
%%%% 计算扰动观测值
iiuav = 5;
d_dw_hat_5 = (lam2w(:) ./ p1w(:)) .* (sig_x1_tilt_1_vec(:,iiuav) + sig_x1_tilt_4_vec(:,iiuav) + sig_x1_tilt_5_vec(:,iiuav));

== matlab function sim_att_dist_obs_tie_2025/cal error dw_tilt ==
  data: dw_vec input; dw_hat_vec input; dw_tilt_vec output
function dw_tilt_vec = fcn(dw_vec, dw_hat_vec)
%%%% 计算扰动观测误差dw_tilt
dw_tilt_vec = zeros(3,5);
for iiuav = 1:5
    dw_tilt_vec(:,iiuav) = dw_vec(:,iiuav) - dw_hat_vec(:,iiuav);
end

== matlab function sim_att_dist_obs_tie_2025/cal sig_x1_tilt agent 1 ==
  data: sig_x1_tilt_1_1 output; x1_tilt_vec input; x1_tilt_squ_1_1 input; sig_x1_tilt_2_1 output; x1_tilt_squ_2_1 input; sig_x1_tilt_3_1 output
function [sig_x1_tilt_1_1, sig_x1_tilt_2_1, sig_x1_tilt_3_1] = fcn(x1_tilt_vec, x1_tilt_squ_1_1, x1_tilt_squ_2_1)
%%%% 计算平滑递增函数
iiuav = 1;
sig_x1_tilt_1_1 = x1_tilt_vec(:,iiuav) .* sign(x1_tilt_vec(:,iiuav));
sig_x1_tilt_2_1 = x1_tilt_squ_1_1(:) .* sign(x1_tilt_vec(:,iiuav));
sig_x1_tilt_3_1 = x1_tilt_squ_2_1(:) .* sign(x1_tilt_vec(:,iiuav));

== matlab function sim_att_dist_obs_tie_2025/choose ksi_est_err 11 ==
  data: x input; y output
function y = fcn(x)
iiuav = 1;
y = x(:,iiuav);

== matlab function sim_att_dist_obs_tie_2025/choose ksi_est_err 12 ==
  data: x input; y output
function y = fcn(x)
iiuav = 1;
y = x(:,iiuav);

== matlab function sim_att_dist_obs_tie_2025/combine dw_hat ==
  data: dw_hat_1 input; dw_hat_2 input; dw_hat_3 input; dw_hat_4 input; dw_hat_5 input; dw_hat_vec output
function dw_hat_vec  = fcn(dw_hat_1, dw_hat_2, dw_hat_3, dw_hat_4, dw_hat_5)
%%%% 合并扰动观测值dw_hat
dw_hat_vec = [dw_hat_1(:), dw_hat_2(:), dw_hat_3(:), dw_hat_4(:), dw_hat_5(:)];

== matlab function sim_att_dist_obs_tie_2025/combine sig_x1_tilt ==
  data: sig_x1_tilt_1_1 input; sig_x1_tilt_1_2 input; sig_x1_tilt_1_3 input; sig_x1_tilt_1_4 input; sig_x1_tilt_1_5 input; sig_x1_tilt_1_vec output; sig_x1_tilt_2_1 input; sig_x1_tilt_2_vec output; sig_x1_tilt_2_2 input; sig_x1_tilt_2_3 input; sig_x1_tilt_2_4 input; sig_x1_tilt_2_5 input; sig_x1_tilt_3_1 input; sig_x1_tilt_3_2 input; sig_x1_tilt_3_3 input; sig_x1_tilt_3_4 input; sig_x1_tilt_3_5 input; sig_x1_tilt_3_vec output
function [sig_x1_tilt_1_vec, sig_x1_tilt_2_vec, sig_x1_tilt_3_vec]  = fcn(sig_x1_tilt_1_1, sig_x1_tilt_1_2, sig_x1_tilt_1_3, sig_x1_tilt_1_4, sig_x1_tilt_1_5, ...
                                                                                                                                sig_x1_tilt_2_1, sig_x1_tilt_2_2, sig_x1_tilt_2_3, sig_x1_tilt_2_4, sig_x1_tilt_2_5, ...
                                                                                                                                sig_x1_tilt_3_1, sig_x1_tilt_3_2, sig_x1_tilt_3_3, sig_x1_tilt_3_4, sig_x1_tilt_3_5)
%%%% 合并领导者位置观测器输出结果
sig_x1_tilt_1_vec = [sig_x1_tilt_1_1(:), sig_x1_tilt_1_2(:), sig_x1_tilt_1_3(:), sig_x1_tilt_1_4(:), sig_x1_tilt_1_5(:)];
sig_x1_tilt_2_vec = [sig_x1_tilt_2_1(:), sig_x1_tilt_2_2(:), sig_x1_tilt_2_3(:), sig_x1_tilt_2_4(:), sig_x1_tilt_2_5(:)];
sig_x1_tilt_3_vec = [sig_x1_tilt_3_1(:), sig_x1_tilt_3_2(:), sig_x1_tilt_3_3(:), sig_x1_tilt_3_4(:), sig_x1_tilt_3_5(:)];

== matlab function sim_att_dist_obs_tie_2025/trans to column51 ==
  data: x input; y output
function y = fcn(x)
y = x(:);

== matlab function sim_att_dist_obs_tie_2025/trans to column52 ==
  data: x input; y output
function y = fcn(x)
y = x(:);

== matlab function sim_att_dist_obs_tie_2025/leader control input ==
  data: t input; u0 output; T1 input; T2 input; R0 input; R1 input; Rx2 input; Ry2 input; Rz2 input
function u0  = fcn(t, T1, T2, R0, R1, Rx2, Ry2, Rz2)
%%%% 给出领导者参考加速度控制输入
u0 = zeros(3, 1);

if t <= ( T1 + 1e-05 )
    u0(1, 1) = - ( 4 * pi * sin( ( 2 * pi * ( t - 0 ) ) / ( 0 - T1 ) ) * ( R0 - R1 ) ) / ( ( 0 - T1 ) ^ 2 ) ...
                        - ( 4 * ( pi ^ 2 ) * cos( ( 2 * pi * ( t - 0 ) ) / ( 0 - T1 ) ) ...
                        * ( R0 + ( ( R0 - R1 ) * ( t - 0 ) ) / ( 0 - T1 ) ) ) / ( ( 0 - T1 ) ^ 2 );
    u0(2, 1) = ( 4 * pi * cos( ( 2 * pi * ( t - 0 ) ) / ( 0 - T1 ) ) * ( R0 - R1 ) ) / ( ( 0 - T1 ) ^ 2 ) ...
                        - ( 4 * ( pi ^ 2 ) * sin( ( 2 * pi * ( t - 0 ) ) / ( 0 - T1 ) ) ...
                        * ( R0 + ( ( R0 - R1 ) * ( t - 0 ) ) / ( 0 - T1 ) ) ) / ( ( 0 - T1 ) ^ 2 );
    u0(3, 1) = 0;
else
    u0(1, 1) = ( 4 * Rx2 * ( pi ^ 2 ) * cos( ( 2 * pi * ( t - T1 ) ) / ( T1 - T2 ) ) ) / ( ( T1 - T2 ) ^ 2 );
    u0(2, 1) = - ( 16 * Ry2 * ( pi ^ 2 ) * sin( ( 4 * pi * ( t - T1 ) ) / ( T1 - T2 ) ) ) / ( ( T1 - T2 ) ^ 2 );
    u0(3, 1) = ( 16 * Rz2 * ( pi ^ 2 ) * sin( ( 4 * pi * ( t - T1 ) ) / ( T1 - T2 ) ) ) / ( ( T1 - T2 ) ^ 2 );
end

== matlab function sim_att_dist_obs_tie_2025/Qei dynam agent 3 ==
  data: Qei_vec input; dQei_3 output; wei_vec input
function dQei_3 = fcn(Qei_vec, wei_vec)
%%%% 更新四元数误差微分方程
iiuav = 3;

wei = wei_vec(:,iiuav);
thetaei = Qei_vec(1,iiuav);
qei = Qei_vec(2:4,iiuav);

GammaQei = zeros(4,3);
GammaQei(1,:) = -(qei');
GammaQei(2:4,:) = thetaei*eye(3,3) + cal_askew_mat(qei);
dQei_3 = (1/2)*GammaQei*wei;

end

== matlab function sim_att_dist_obs_tie_2025/Qei dynam agent 4 ==
  data: Qei_vec input; dQei_4 output; wei_vec input
function dQei_4 = fcn(Qei_vec, wei_vec)
%%%% 更新四元数误差微分方程
iiuav = 4;

wei = wei_vec(:,iiuav);
thetaei = Qei_vec(1,iiuav);
qei = Qei_vec(2:4,iiuav);

GammaQei = zeros(4,3);
GammaQei(1,:) = -(qei');
GammaQei(2:4,:) = thetaei*eye(3,3) + cal_askew_mat(qei);
dQei_4 = (1/2)*GammaQei*wei;

end

== matlab function sim_att_dist_obs_tie_2025/Qei dynam agent 5 ==
  data: Qei_vec input; dQei_5 output; wei_vec input
function dQei_5 = fcn(Qei_vec, wei_vec)
%%%% 更新四元数误差微分方程
iiuav = 5;

wei = wei_vec(:,iiuav);
thetaei = Qei_vec(1,iiuav);
qei = Qei_vec(2:4,iiuav);

GammaQei = zeros(4,3);
GammaQei(1,:) = -(qei');
GammaQei(2:4,:) = thetaei*eye(3,3) + cal_askew_mat(qei);
dQei_5 = (1/2)*GammaQei*wei;

end

== matlab function sim_att_dist_obs_tie_2025/Qi dynam agent 1 ==
  data: Qi_vec input; dQi_1 output; wi_vec input
function dQi_1 = fcn(Qi_vec, wi_vec)
%%%% 更新四元数微分方程
iiuav = 1;

wi = wi_vec(:,iiuav);
thetai = Qi_vec(1,iiuav);
qi = Qi_vec(2:4,iiuav);

GammaQi = zeros(4,3);
GammaQi(1,:) = -(qi');
GammaQi(2:4,:) = thetai*eye(3,3) + cal_askew_mat(qi);
dQi_1 = (1/2)*GammaQi*wi;

end

== matlab function sim_att_dist_obs_tie_2025/Qi dynam agent 2 ==
  data: Qi_vec input; dQi_2 output; wi_vec input
function dQi_2 = fcn(Qi_vec, wi_vec)
%%%% 更新四元数微分方程
iiuav = 2;

wi = wi_vec(:,iiuav);
thetai = Qi_vec(1,iiuav);
qi = Qi_vec(2:4,iiuav);

GammaQi = zeros(4,3);
GammaQi(1,:) = -(qi');
GammaQi(2:4,:) = thetai*eye(3,3) + cal_askew_mat(qi);
dQi_2 = (1/2)*GammaQi*wi;

end

== matlab function sim_att_dist_obs_tie_2025/Qi dynam agent 3 ==
  data: Qi_vec input; dQi_3 output; wi_vec input
function dQi_3 = fcn(Qi_vec, wi_vec)
%%%% 更新四元数微分方程
iiuav = 3;

wi = wi_vec(:,iiuav);
thetai = Qi_vec(1,iiuav);
qi = Qi_vec(2:4,iiuav);

GammaQi = zeros(4,3);
GammaQi(1,:) = -(qi');
GammaQi(2:4,:) = thetai*eye(3,3) + cal_askew_mat(qi);
dQi_3 = (1/2)*GammaQi*wi;

end

== matlab function sim_att_dist_obs_tie_2025/Qi dynam agent 4 ==
  data: Qi_vec input; dQi_4 output; wi_vec input
function dQi_4 = fcn(Qi_vec, wi_vec)
%%%% 更新四元数微分方程
iiuav = 4;

wi = wi_vec(:,iiuav);
thetai = Qi_vec(1,iiuav);
qi = Qi_vec(2:4,iiuav);

GammaQi = zeros(4,3);
GammaQi(1,:) = -(qi');
GammaQi(2:4,:) = thetai*eye(3,3) + cal_askew_mat(qi);
dQi_4 = (1/2)*GammaQi*wi;

end

== matlab function sim_att_dist_obs_tie_2025/Qi dynam agent 5 ==
  data: Qi_vec input; dQi_5 output; wi_vec input
function dQi_5 = fcn(Qi_vec, wi_vec)
%%%% 更新四元数微分方程
iiuav = 5;

wi = wi_vec(:,iiuav);
thetai = Qi_vec(1,iiuav);
qi = Qi_vec(2:4,iiuav);

GammaQi = zeros(4,3);
GammaQi(1,:) = -(qi');
GammaQi(2:4,:) = thetai*eye(3,3) + cal_askew_mat(qi);
dQi_5 = (1/2)*GammaQi*wi;

end

== matlab function sim_att_dist_obs_tie_2025/cal Fi_S agent 1 ==
  data: cS0 input; Ji input; wi_vec input; wci_vec input; wei_vec input; Fi_S_1 output; dwci_vec input; Rei_vec input; Phi_bar_psi_e_vec input
function Fi_S_1 = fcn(cS0, Ji, wi_vec, wci_vec, wei_vec, dwci_vec, Rei_vec, Phi_bar_psi_e_vec)
%%%% 计算补偿项
iiuav = 1;
Fi_S_1 = -cal_askew_mat( wi_vec(:,iiuav) ) * Ji(:,:,iiuav) * wi_vec(:,iiuav) ...
                + Ji(:,:,iiuav) * cal_askew_mat( wei_vec(:,iiuav) ) * ( Rei_vec(:,:,iiuav)' ) * wci_vec(:,iiuav) ...
                - Ji(:,:,iiuav) * ( Rei_vec(:,:,iiuav)' ) * dwci_vec(:,iiuav) ...
                + cS0 * Ji(:,:,iiuav) * Phi_bar_psi_e_vec(:,iiuav);

== matlab function sim_att_dist_obs_tie_2025/cal Fi_S agent 2 ==
  data: cS0 input; Ji input; wi_vec input; wci_vec input; wei_vec input; Fi_S_2 output; dwci_vec input; Rei_vec input; Phi_bar_psi_e_vec input
function Fi_S_2 = fcn(cS0, Ji, wi_vec, wci_vec, wei_vec, dwci_vec, Rei_vec, Phi_bar_psi_e_vec)
%%%% 计算补偿项
iiuav = 2;
Fi_S_2 = -cal_askew_mat( wi_vec(:,iiuav) ) * Ji(:,:,iiuav) * wi_vec(:,iiuav) ...
                + Ji(:,:,iiuav) * cal_askew_mat( wei_vec(:,iiuav) ) * ( Rei_vec(:,:,iiuav)' ) * wci_vec(:,iiuav) ...
                - Ji(:,:,iiuav) * ( Rei_vec(:,:,iiuav)' ) * dwci_vec(:,iiuav) ...
                + cS0 * Ji(:,:,iiuav) * Phi_bar_psi_e_vec(:,iiuav);

== matlab function sim_att_dist_obs_tie_2025/cal Fi_S agent 3 ==
  data: cS0 input; Ji input; wi_vec input; wci_vec input; wei_vec input; Fi_S_3 output; dwci_vec input; Rei_vec input; Phi_bar_psi_e_vec input
function Fi_S_3 = fcn(cS0, Ji, wi_vec, wci_vec, wei_vec, dwci_vec, Rei_vec, Phi_bar_psi_e_vec)
%%%% 计算补偿项
iiuav = 3;
Fi_S_3 = -cal_askew_mat( wi_vec(:,iiuav) ) * Ji(:,:,iiuav) * wi_vec(:,iiuav) ...
                + Ji(:,:,iiuav) * cal_askew_mat( wei_vec(:,iiuav) ) * ( Rei_vec(:,:,iiuav)' ) * wci_vec(:,iiuav) ...
                - Ji(:,:,iiuav) * ( Rei_vec(:,:,iiuav)' ) * dwci_vec(:,iiuav) ...
                + cS0 * Ji(:,:,iiuav) * Phi_bar_psi_e_vec(:,iiuav);

== matlab function sim_att_dist_obs_tie_2025/cal Fi_S agent 4 ==
  data: cS0 input; Ji input; wi_vec input; wci_vec input; wei_vec input; Fi_S_4 output; dwci_vec input; Rei_vec input; Phi_bar_psi_e_vec input
function Fi_S_4 = fcn(cS0, Ji, wi_vec, wci_vec, wei_vec, dwci_vec, Rei_vec, Phi_bar_psi_e_vec)
%%%% 计算补偿项
iiuav = 4;
Fi_S_4 = -cal_askew_mat( wi_vec(:,iiuav) ) * Ji(:,:,iiuav) * wi_vec(:,iiuav) ...
                + Ji(:,:,iiuav) * cal_askew_mat( wei_vec(:,iiuav) ) * ( Rei_vec(:,:,iiuav)' ) * wci_vec(:,iiuav) ...
                - Ji(:,:,iiuav) * ( Rei_vec(:,:,iiuav)' ) * dwci_vec(:,iiuav) ...
                + cS0 * Ji(:,:,iiuav) * Phi_bar_psi_e_vec(:,iiuav);

== matlab function sim_att_dist_obs_tie_2025/cal Fi_S agent 5 ==
  data: cS0 input; Ji input; wi_vec input; wci_vec input; wei_vec input; Fi_S_5 output; dwci_vec input; Rei_vec input; Phi_bar_psi_e_vec input
function Fi_S_5 = fcn(cS0, Ji, wi_vec, wci_vec, wei_vec, dwci_vec, Rei_vec, Phi_bar_psi_e_vec)
%%%% 计算补偿项
iiuav = 5;
Fi_S_5 = -cal_askew_mat( wi_vec(:,iiuav) ) * Ji(:,:,iiuav) * wi_vec(:,iiuav) ...
                + Ji(:,:,iiuav) * cal_askew_mat( wei_vec(:,iiuav) ) * ( Rei_vec(:,:,iiuav)' ) * wci_vec(:,iiuav) ...
                - Ji(:,:,iiuav) * ( Rei_vec(:,:,iiuav)' ) * dwci_vec(:,iiuav) ...
                + cS0 * Ji(:,:,iiuav) * Phi_bar_psi_e_vec(:,iiuav);

== matlab function sim_att_dist_obs_tie_2025/cal Phi_bar_psi_e agent 1 ==
  data: pp0 input; Phi_bar_psi_e_node_1 output; beta_Phi_1 input; beta_Phi_2 input; thr_p_plus_1 input; gamma0 input; eps_s_bar_div_pi input; wei_vec input; S_bar_vec input; V_Phi_Rei_div_pi_vec input; V_Phi_Rei_squ_p_min_1_vec input; V_Phi_Rei_squ_p_plus_1_vec input; V_Phi_Rei_squ_2p_vec input
function Phi_bar_psi_e_node_1 = fcn(pp0, beta_Phi_1, beta_Phi_2, thr_p_plus_1, gamma0, ...
                                                                    eps_s_bar_div_pi, wei_vec, S_bar_vec, V_Phi_Rei_div_pi_vec, ...
                                                                    V_Phi_Rei_squ_p_min_1_vec, V_Phi_Rei_squ_p_plus_1_vec, V_Phi_Rei_squ_2p_vec)
%%%% 计算姿态误差项
iiuav = 1;
Phi_bar_psi_e_node_1 = zeros(3,1);
for kk = 1:3
    if S_bar_vec(kk, iiuav) == 0
        Phi_bar_psi_e_node_1(kk, 1) = thr_p_plus_1 * ( pp0 + 1 ) * V_Phi_Rei_div_pi_vec(kk, iiuav) ...
                                                                * V_Phi_Rei_squ_p_min_1_vec(kk, iiuav) * wei_vec(kk, iiuav) ...
                                                                / ( 2 * tanh( ( gamma0 / 2 ) * V_Phi_Rei_div_pi_vec(kk, iiuav) ) ) ...
                                                                + ( thr_p_plus_1 * gamma0 / 4 ) * V_Phi_Rei_squ_p_plus_1_vec(kk, iiuav) ...
                                                                * ( ( sech( ( gamma0 / 2 ) * V_Phi_Rei_div_pi_vec(kk, iiuav) ) ...
                                                                / tanh( ( gamma0 / 2 ) * V_Phi_Rei_div_pi_vec(kk, iiuav) ) ) ^ 2 ) * wei_vec(kk, iiuav);
    else
        if abs( V_Phi_Rei_div_pi_vec ) > eps_s_bar_div_pi
            Phi_bar_psi_e_node_1(kk, 1) = thr_p_plus_1 * ( pp0 + 1 ) * V_Phi_Rei_div_pi_vec(kk, iiuav) ...
                                                                    * V_Phi_Rei_squ_p_min_1_vec(kk, iiuav) * wei_vec(kk, iiuav) ...
                                                                    / ( 2 * tanh( ( gamma0 / 2 ) * V_Phi_Rei_div_pi_vec(kk, iiuav) ) ) ...
                                                                    + ( thr_p_plus_1 * gamma0 / 4 ) * V_Phi_Rei_squ_p_plus_1_vec(kk, iiuav) ...
                                                                    * ( ( sech( ( gamma0 / 2 ) * V_Phi_Rei_div_pi_vec(kk, iiuav) ) ...
                                                                    / tanh( ( gamma0 / 2 ) * V_Phi_Rei_div_pi_vec(kk, iiuav) ) ) ^ 2 ) * wei_vec(kk, iiuav);
        else
            Phi_bar_psi_e_node_1(kk, 1) = 2 * beta_Phi_1 * ( ( abs( V_Phi_Rei_div_pi_vec(kk, iiuav) ) ) ^ 2 ) * wei_vec(kk, iiuav) ...
                                                                    + ( 2 * pp0 + 1 ) * beta_Phi_2 * V_Phi_Rei_squ_2p_vec(kk, iiuav) * wei_vec(kk, iiuav);
        end
    end
end
